simulink model "BulkModulus"  (Simulink 8.5)
settings: Solver=ode4  StartTime=0.0  StopTime=10.0  FixedStep=sampleTime  RelTol=1e-3
undefined symbols (not defined in the file): Be, gamma_air, Sel_bulk, Sel_ent_air
settings Model: Creator=HBALLEST  LastModifiedBy=Pedro H  SimulationMode=accelerator
settings DataIOCC: SignalLoggingSaveFormat=Dataset
settings OptimizationCC: InlineParams=on
settings DebuggingCC: UnderspecifiedInitializationDetection=Simplified  MergeDetectMultiDrivingBlocksExec=error  FcnCallInpInsideContextMsg=EnableAllAsError
settings ModelReferenceCC: UpdateModelReferenceTargets=IfOutOfDate
settings GRTTargetCC: CombineOutputUpdateFcns=on  GRTInterface=off

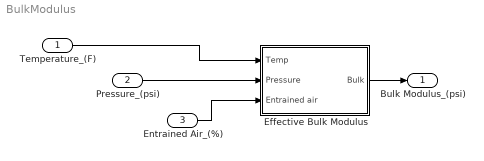
== system BulkModulus ==
  Temperature_(F) : Inport
  Pressure_(psi) : Inport  Port=2
  Entrained Air_(%) : Inport  Port=3
  Effective Bulk Modulus : Subsystem
  Bulk Modulus_(psi) : Outport
  wires:
  Effective Bulk Modulus/1(Bulk) -> Bulk Modulus_(psi)/1
  Temperature_(F)/1 -> Effective Bulk Modulus/1(Temp)
  Pressure_(psi)/1 -> Effective Bulk Modulus/2(Pressure)
  Entrained Air_(%)/1 -> Effective Bulk Modulus/3(Entrained air)

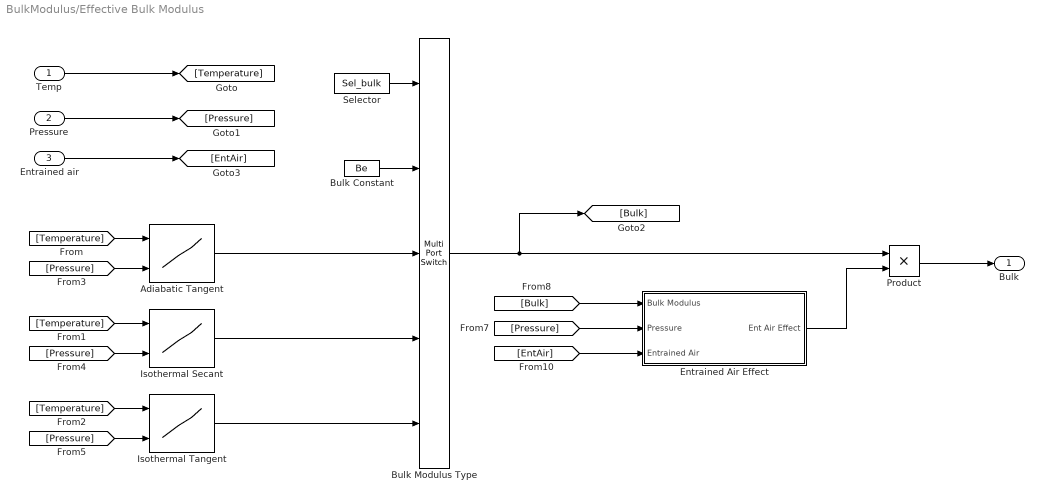
== system BulkModulus/Effective Bulk Modulus ==
  Temp : Inport
  Pressure : Inport  Port=2
  Entrained air : Inport  Port=3
  Adiabatic Tangent : Lookup_n-D  BreakpointsForDimension1=[0:10:200]  BreakpointsForDimension2=[1500 3000 5000 8000]  Table=|  RndMeth=Simplest  InputSameDT=on
      | [[328385
      | 317493
      | 306938
      | 296717
      | 286828
      | 277269
      | 268038
      | 259133
      | 250552
      | 242293
      | 234353
      | 226730
      | 219423
      | 212429
      | 205746
      | 199373
      | 193306
      | 187544
      | 182084
      | 176925
      | 172064
      | ],[457660
      | 438564
      | 420172
      | 402478
      | 385479
      | 369170
      | 353546
      | 338602
      | 324335
      | 310740
      | 297812
      | 285547
      | 273940
      | 262986
      | 252681
      | 243021
      | 234001
      | 225616
      | 217863
      | 210735
      | 204230
      | ],[461068
      | 445006
      | 429505
      | 414562
      | 400174
      | 386337
      | 373047
      | 360301
      | 348095
      | 336426
      | 325289
      | 314682
      | 304600
      | 295041
      | 286000
      | 277474
      | 269459
      | 261952
      | 254949
      | 248447
      | 242442
      | ],[531133
      | 516205
      | 501737
      | 487727
      | 474171
      | 461068
      | 448414
      | 436206
      | 424442
      | 413117
      | 402230
      | 391778
      | 381757
      | 372166
      | 363000
      | 354256
      | 345933
      | 338028
      | 330536
      | 323456
      | 316784
      | ]]
  Bulk Constant : Constant  Value=Be
  Bulk Modulus Type : MultiPortSwitch  Inputs=4
  Entrained Air Effect : Subsystem
  Isothermal Secant : Lookup_n-D  BreakpointsForDimension1=[0:10:200]  BreakpointsForDimension2=[0 1500 3000]  Table=|  RndMeth=Simplest  InputSameDT=on
      | [[251501
      | 242817
      | 234410
      | 226279
      | 218424
      | 210846
      | 203544
      | 196518
      | 189768
      | 183295
      | 177098
      | 171177
      | 165533
      | 160165
      | 155073
      | 150257
      | 145718
      | 141455
      | 137468
      | 133757
      | 130323],[259556
      | 251093
      | 242886
      | 234934
      | 227239
      | 219798
      | 212614
      | 205685
      | 199012
      | 192594
      | 186433
      | 180526
      | 174876
      | 169481
      | 164342
      | 159458
      | 154831
      | 150458
      | 146342
      | 142481
      | 138876
      | ],[267611
      | 259369
      | 251362
      | 243590
      | 236053
      | 228751
      | 221684
      | 214852
      | 208255
      | 201894
      | 195767
      | 189875
      | 184219
      | 178797
      | 173611
      | 168660
      | 163943
      | 159462
      | 155216
      | 151205
      | 147429]]
  Isothermal Tangent : Lookup_n-D  BreakpointsForDimension1=[0:10:200]  BreakpointsForDimension2=[0 1500 3000 8000]  Table=|  RndMeth=Simplest  InputSameDT=on
      | [[267611
      | 259369
      | 251362
      | 243590
      | 236053
      | 228751
      | 221684
      | 214852
      | 208255
      | 201894
      | 195767
      | 189875
      | 184219
      | 178797
      | 173611
      | 168660
      | 163943
      | 159462
      | 155216
      | 151205
      | 147429],[372961
      | 358275
      | 344093
      | 330415
      | 317241
      | 304570
      | 292404
      | 280742
      | 269583
      | 258929
      | 248778
      | 239131
      | 229989
      | 221350
      | 213215
      | 205584
      | 198457
      | 191834
      | 185715
      | 180100
      | 174989],[375738
      | 363537
      | 351736
      | 340335
      | 329334
      | 318734
      | 308533
      | 298732
      | 289332
      | 280331
      | 271731
      | 263531
      | 255730
      | 248330
      | 241330
      | 234730
      | 228530
      | 222730
      | 217330
      | 212330
      | 207730],[432836
      | 421701
      | 410889
      | 400400
      | 390232
      | 380388
      | 370866
      | 361667
      | 352790
      | 344236
      | 336004
      | 328095
      | 320508
      | 313244
      | 306303
      | 299684
      | 293388
      | 287414
      | 281763
      | 276434
      | 271428]]
  Product : Product  RndMeth=Zero
  Selector : Constant  Value=Sel_bulk
  Bulk : Outport
  wires:
  Bulk Modulus Type/1 -> [Bulk], Product/1
  Selector/1 -> Bulk Modulus Type/1
  Isothermal Tangent/1 -> Bulk Modulus Type/5
  Isothermal Secant/1 -> Bulk Modulus Type/4
  Bulk Constant/1 -> Bulk Modulus Type/2
  Adiabatic Tangent/1 -> Bulk Modulus Type/3
  Temp/1 -> [Temperature]
  [Temperature] -> Adiabatic Tangent/1
  [Temperature] -> Isothermal Secant/1
  [Temperature] -> Isothermal Tangent/1
  Pressure/1 -> [Pressure]
  [Pressure] -> Adiabatic Tangent/2
  [Pressure] -> Isothermal Secant/2
  [Pressure] -> Isothermal Tangent/2
  [Pressure] -> Entrained Air Effect/2(Pressure)
  Entrained Air Effect/1(Ent Air Effect) -> Product/2
  [Bulk] -> Entrained Air Effect/1(Bulk Modulus)
  Entrained air/1 -> [EntAir]
  [EntAir] -> Entrained Air Effect/3(Entrained Air)
  Product/1 -> Bulk/1

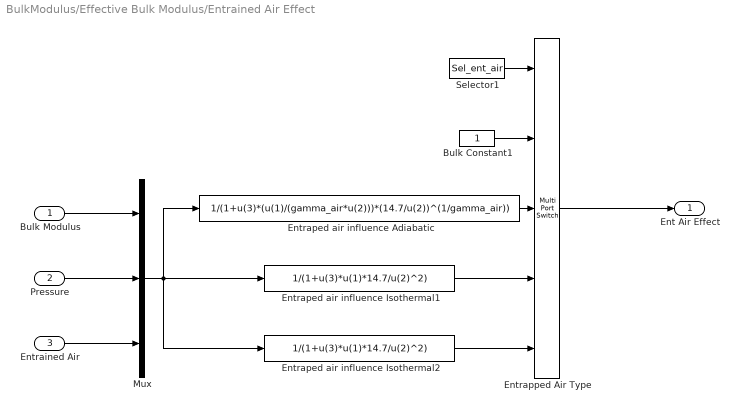
== system BulkModulus/Effective Bulk Modulus/Entrained Air Effect ==
  Bulk Modulus : Inport
  Pressure : Inport  Port=2
  Entrained Air : Inport  Port=3
  Bulk Constant1 : Constant
  Entraped air influence Adiabatic : Fcn  Expr=1/(1+u(3)*(u(1)/(gamma_air*u(2)))*(14.7/u(2))^(1/gamma_air))
  Entraped air influence Isothermal1 : Fcn  Expr=1/(1+u(3)*u(1)*14.7/u(2)^2)
  Entraped air influence Isothermal2 : Fcn  Expr=1/(1+u(3)*u(1)*14.7/u(2)^2)
  Entrapped Air Type : MultiPortSwitch  Inputs=4
  Mux : Mux  Inputs=3
  Selector1 : Constant  Value=Sel_ent_air
  Ent Air Effect : Outport
  wires:
  Entrapped Air Type/1 -> Ent Air Effect/1
  Bulk Constant1/1 -> Entrapped Air Type/2
  Entraped air influence Adiabatic/1 -> Entrapped Air Type/3
  Entraped air influence Isothermal2/1 -> Entrapped Air Type/5
  Entraped air influence Isothermal1/1 -> Entrapped Air Type/4
  Selector1/1 -> Entrapped Air Type/1
  Mux/1 -> Entraped air influence Isothermal1/1, Entraped air influence Adiabatic/1, Entraped air influence Isothermal2/1
  Bulk Modulus/1 -> Mux/1
  Pressure/1 -> Mux/2
  Entrained Air/1 -> Mux/3
